simulink library "voting_scheme_lib"  (R2018b)
settings: Solver=VariableStepAuto  StartTime=0.0  StopTime=10.0  RelTol=1e-3
undefined symbols (not defined in the file): simParams
libraries: dspindex x4, FSW_Lib x1, aerolibutil x1
settings Model: Creator=devantormey  LastModifiedBy=kylle

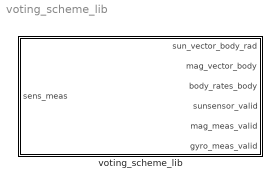
== system voting_scheme_lib ==
  voting_scheme_lib : Subsystem

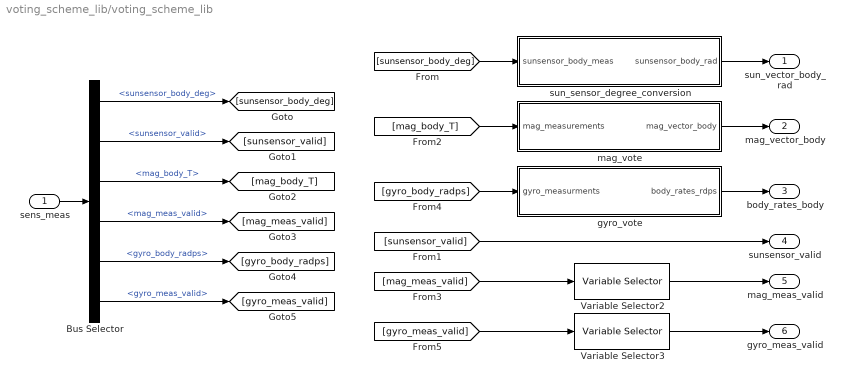
== system voting_scheme_lib/voting_scheme_lib ==
  sens_meas : Inport
  Bus Selector : BusSelector  OutputSignals=sunsensor_body_deg,sunsensor_valid,mag_body_T,mag_meas_valid,gyro_body_radps,gyro_meas_valid
  Variable Selector2 : dspindex/Variable Selector  NumInputs=1  rowsOrCols=Rows  IdxMode=Fixed  Elements=[1]  ZerOneIdxMode=One-based  errmode=Clip Index  FillMode=off  FillValues=0
  Variable Selector3 : dspindex/Variable Selector  NumInputs=1  rowsOrCols=Rows  IdxMode=Fixed  Elements=[1]  ZerOneIdxMode=One-based  errmode=Clip Index  FillMode=off  FillValues=0
  gyro_vote : Subsystem
  mag_vote : Subsystem
  sun_sensor_degree_conversion : Subsystem
  sun_vector_body_rad : Outport
  mag_vector_body : Outport  Port=2
  body_rates_body : Outport  Port=3
  sunsensor_valid : Outport  Port=4
  mag_meas_valid : Outport  Port=5
  gyro_meas_valid : Outport  Port=6
  wires:
  Variable Selector3/1 -> gyro_meas_valid/1
  [gyro_meas_valid] -> Variable Selector3/1
  Variable Selector2/1 -> mag_meas_valid/1
  [mag_meas_valid] -> Variable Selector2/1
  [sunsensor_valid] -> sunsensor_valid/1
  Bus Selector/6 -> [gyro_meas_valid]  "<gyro_meas_valid>"
  Bus Selector/5 -> [gyro_body_radps]  "<gyro_body_radps>"
  Bus Selector/4 -> [mag_meas_valid]  "<mag_meas_valid>"
  Bus Selector/3 -> [mag_body_T]  "<mag_body_T>"
  Bus Selector/2 -> [sunsensor_valid]  "<sunsensor_valid>"
  [sunsensor_body_deg] -> sun_sensor_degree_conversion/1(sunsensor_body_meas)
  Bus Selector/1 -> [sunsensor_body_deg]  "<sunsensor_body_deg>"
  mag_vote/1(mag_vector_body) -> mag_vector_body/1
  [mag_body_T] -> mag_vote/1(mag_measurements)
  sun_sensor_degree_conversion/1(sunsensor_body_rad) -> sun_vector_body_rad/1
  [gyro_body_radps] -> gyro_vote/1(gyro_measurments)
  gyro_vote/1(body_rates_rdps) -> body_rates_body/1
  sens_meas/1 -> Bus Selector/1

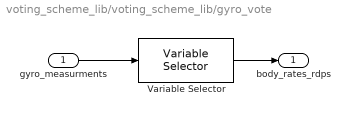
== system voting_scheme_lib/voting_scheme_lib/gyro_vote ==
  gyro_measurments : Inport
  Variable Selector : dspindex/Variable Selector  NumInputs=1  rowsOrCols=Columns  IdxMode=Fixed  Elements=[1]  ZerOneIdxMode=One-based  errmode=Clip Index  FillMode=off  FillValues=0
  body_rates_rdps : Outport
  wires:
  gyro_measurments/1 -> Variable Selector/1
  Variable Selector/1 -> body_rates_rdps/1

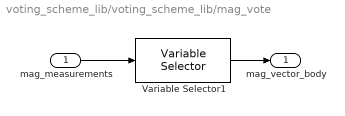
== system voting_scheme_lib/voting_scheme_lib/mag_vote ==
  mag_measurements : Inport
  Variable Selector1 : dspindex/Variable Selector  NumInputs=1  rowsOrCols=Columns  IdxMode=Fixed  Elements=[1]  ZerOneIdxMode=One-based  errmode=Clip Index  FillMode=off  FillValues=0
  mag_vector_body : Outport
  wires:
  Variable Selector1/1 -> mag_vector_body/1
  mag_measurements/1 -> Variable Selector1/1

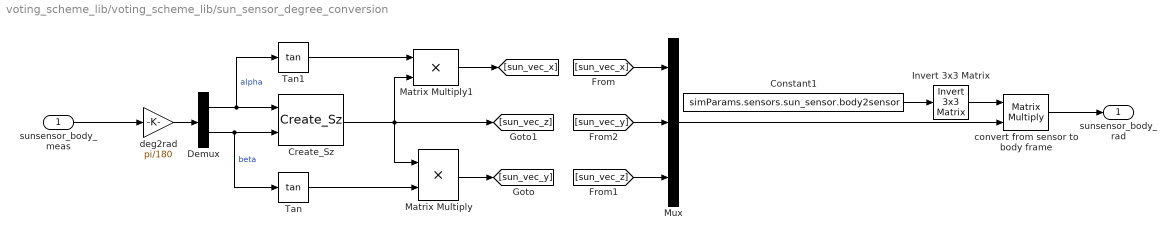
== system voting_scheme_lib/voting_scheme_lib/sun_sensor_degree_conversion ==
  sunsensor_body_meas : Inport
  Constant1 : Constant  Value=simParams.sensors.sun_sensor.body2sensor
  Create_Sz : FSW_Lib/FSW_Lib/Conversion_lib/sunsensor_body_deg2rad/Create_Sz  SystemSampleTime=-1
  Demux : Demux  Outputs=2
  Invert 3x3 Matrix : aerolibutil/Invert  3x3 Matrix
  Matrix Multiply : Product
  Matrix Multiply1 : Product
  Mux : Mux  Inputs=3
  Tan : Trigonometry  Operator=tan
  Tan1 : Trigonometry  Operator=tan
  convert from sensor to body frame : Product  Multiplication=Matrix(*)
  deg2rad : Gain  Gain=pi/180
  sunsensor_body_rad : Outport
  wires:
  Constant1/1 -> Invert 3x3 Matrix/1
  [sun_vec_y] -> Mux/2
  sunsensor_body_meas/1 -> deg2rad/1
  Mux/1 -> convert from sensor to body frame/2
  Tan1/1 -> Matrix Multiply1/1
  Demux/2 -> Tan/1, Create_Sz/2  "beta"
  [sun_vec_z] -> Mux/3
  deg2rad/1 -> Demux/1
  [sun_vec_x] -> Mux/1
  Create_Sz/1 -> [sun_vec_z], Matrix Multiply/1, Matrix Multiply1/2
  Invert 3x3 Matrix/1 -> convert from sensor to body frame/1
  Matrix Multiply1/1 -> [sun_vec_x]
  convert from sensor to body frame/1 -> sunsensor_body_rad/1
  Demux/1 -> Tan1/1, Create_Sz/1  "alpha"
  Tan/1 -> Matrix Multiply/2
  Matrix Multiply/1 -> [sun_vec_y]
